simulink model "SVM_Stepper"  (R2020b)
settings: Solver=VariableStepAuto  StartTime=0.0  StopTime=1  FixedStep=0.0001  MaxStep=0.000005  RelTol=1e-3
values from neighbouring files (symbols this model uses):
  b = 0.05    [system_parameters.m]
  J = 48e-6    (= 4.8e-05)    [system_parameters.m]
  K_t = T_hold/I_rms    (= 0.575)    [system_parameters.m]
  L = 2e-3    (= 0.002)    [system_parameters.m]
  p = 50    [system_parameters.m]
  R = 0.5    [system_parameters.m]
  T_dm = 0.068    [system_parameters.m]
  T_load = 5.06e-3    (= 0.00506)    [system_parameters.m]
  U = 24    [system_parameters.m]
undefined symbols (not defined in the file or in its folder): Down, Up
libraries: fl_lib x90, ee_lib x55, eePwmGenerator x37, nesl_utility x33, dspsrcs4 x18, pid_lib x6, powerlib x4, eeDcCurrentController x1, eePmsmTorqueEstimator x1, simulink x1, eeQuadratureDecoder x1
(part 2 of 2)

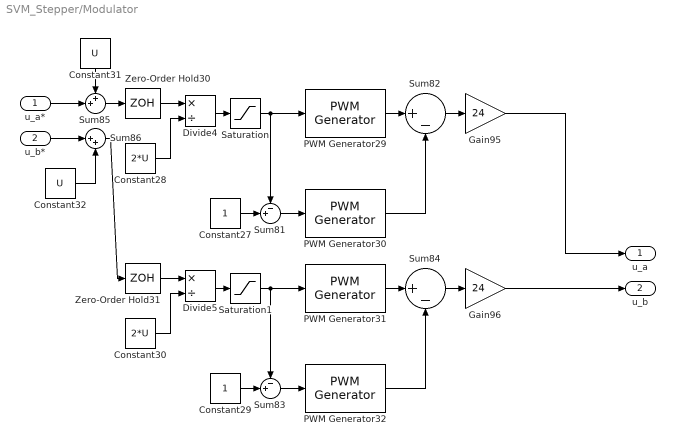
== system SVM_Stepper/Modulator ==
  u_a* : Inport
  u_b* : Inport  Port=2
  Constant27 : Constant
  Constant28 : Constant  Value=2*U
  Constant29 : Constant
  Constant30 : Constant  Value=2*U
  Constant31 : Constant  Value=U
  Constant32 : Constant  Value=U
  Divide4 : Product  Inputs=*/
  Divide5 : Product  Inputs=*/
  Gain95 : Gain  Gain=24
  Gain96 : Gain  Gain=24
  PWM Generator{29..32} (4 alike) : eePwmGenerator/PWM Generator  CarrCount=Up  Tper=25e-6  Ts=1e-6
  Saturation : Saturate  UpperLimit=1  LowerLimit=0
  Saturation1 : Saturate  UpperLimit=1  LowerLimit=0
  Sum81 : Sum  Inputs=-+|
  Sum82 : Sum  Inputs=|+-
  Sum83 : Sum  Inputs=-+|
  Sum84 : Sum  Inputs=|+-
  Sum85 : Sum  Inputs=++|
  Sum86 : Sum  Inputs=|++
  Zero-Order Hold30 : ZeroOrderHold  SampleTime=50e-6
  Zero-Order Hold31 : ZeroOrderHold  SampleTime=50e-6
  u_a : Outport
  u_b : Outport  Port=2
  wires:
  u_a*/1 -> Sum85/2
  Gain96/1 -> u_b/1
  Sum86/1 -> Zero-Order Hold31/1
  Saturation/1 -> PWM Generator29/1, Sum81/1
  Constant32/1 -> Sum86/2
  Zero-Order Hold30/1 -> Divide4/1
  Sum82/1 -> Gain95/1
  PWM Generator29/1 -> Sum82/1
  Constant30/1 -> Divide5/2
  Constant28/1 -> Divide4/2
  PWM Generator31/1 -> Sum84/1
  Saturation1/1 -> PWM Generator31/1, Sum83/1
  Divide4/1 -> Saturation/1
  PWM Generator30/1 -> Sum82/2
  Sum81/1 -> PWM Generator30/1
  Constant27/1 -> Sum81/2
  Constant29/1 -> Sum83/2
  Sum83/1 -> PWM Generator32/1
  Sum84/1 -> Gain96/1
  Divide5/1 -> Saturation1/1
  PWM Generator32/1 -> Sum84/2
  Zero-Order Hold31/1 -> Divide5/1
  Sum85/1 -> Zero-Order Hold30/1
  Constant31/1 -> Sum85/1
  Gain95/1 -> u_a/1
  u_b*/1 -> Sum86/1

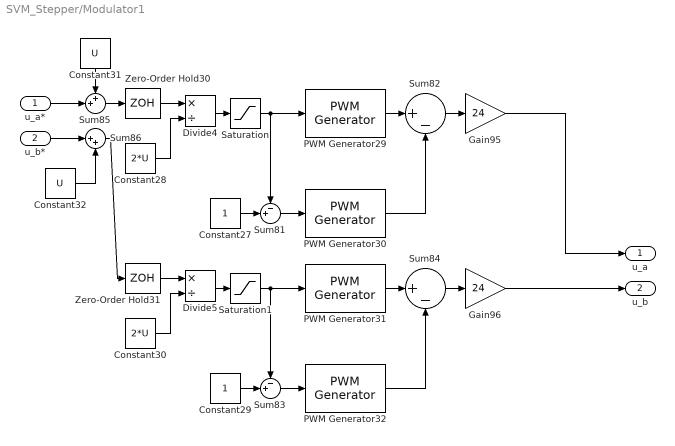
== system SVM_Stepper/Modulator1 ==
  u_a* : Inport
  u_b* : Inport  Port=2
  Constant27 : Constant
  Constant28 : Constant  Value=2*U
  Constant29 : Constant
  Constant30 : Constant  Value=2*U
  Constant31 : Constant  Value=U
  Constant32 : Constant  Value=U
  Divide4 : Product  Inputs=*/
  Divide5 : Product  Inputs=*/
  Gain95 : Gain  Gain=24
  Gain96 : Gain  Gain=24
  PWM Generator{29..32} (4 alike) : eePwmGenerator/PWM Generator  CarrCount=Up  Tper=25e-6  Ts=1e-6
  Saturation : Saturate  UpperLimit=1  LowerLimit=0
  Saturation1 : Saturate  UpperLimit=1  LowerLimit=0
  Sum81 : Sum  Inputs=-+|
  Sum82 : Sum  Inputs=|+-
  Sum83 : Sum  Inputs=-+|
  Sum84 : Sum  Inputs=|+-
  Sum85 : Sum  Inputs=++|
  Sum86 : Sum  Inputs=|++
  Zero-Order Hold30 : ZeroOrderHold  SampleTime=50e-6
  Zero-Order Hold31 : ZeroOrderHold  SampleTime=50e-6
  u_a : Outport
  u_b : Outport  Port=2
  wires:
  u_a*/1 -> Sum85/2
  Gain96/1 -> u_b/1
  Sum86/1 -> Zero-Order Hold31/1
  Saturation/1 -> PWM Generator29/1, Sum81/1
  Constant32/1 -> Sum86/2
  Zero-Order Hold30/1 -> Divide4/1
  Sum82/1 -> Gain95/1
  PWM Generator29/1 -> Sum82/1
  Constant30/1 -> Divide5/2
  Constant28/1 -> Divide4/2
  PWM Generator31/1 -> Sum84/1
  Saturation1/1 -> PWM Generator31/1, Sum83/1
  Divide4/1 -> Saturation/1
  PWM Generator30/1 -> Sum82/2
  Sum81/1 -> PWM Generator30/1
  Constant27/1 -> Sum81/2
  Constant29/1 -> Sum83/2
  Sum83/1 -> PWM Generator32/1
  Sum84/1 -> Gain96/1
  Divide5/1 -> Saturation1/1
  PWM Generator32/1 -> Sum84/2
  Zero-Order Hold31/1 -> Divide5/1
  Sum85/1 -> Zero-Order Hold30/1
  Constant31/1 -> Sum85/1
  Gain95/1 -> u_a/1
  u_b*/1 -> Sum86/1

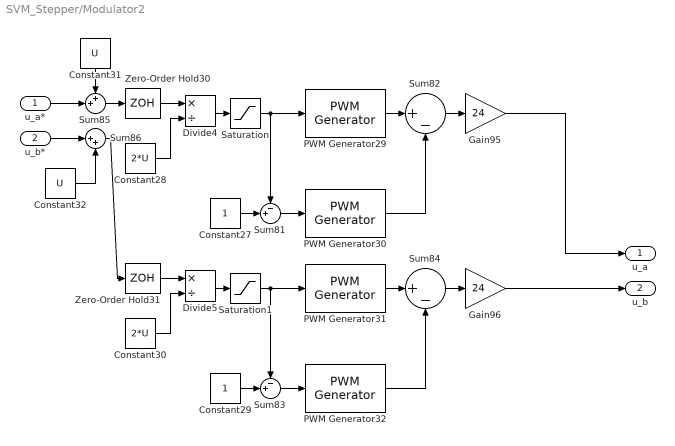
== system SVM_Stepper/Modulator2 ==
  u_a* : Inport
  u_b* : Inport  Port=2
  Constant27 : Constant
  Constant28 : Constant  Value=2*U
  Constant29 : Constant
  Constant30 : Constant  Value=2*U
  Constant31 : Constant  Value=U
  Constant32 : Constant  Value=U
  Divide4 : Product  Inputs=*/
  Divide5 : Product  Inputs=*/
  Gain95 : Gain  Gain=24
  Gain96 : Gain  Gain=24
  PWM Generator{29..32} (4 alike) : eePwmGenerator/PWM Generator  CarrCount=Up  Tper=25e-6  Ts=1e-6
  Saturation : Saturate  UpperLimit=1  LowerLimit=0
  Saturation1 : Saturate  UpperLimit=1  LowerLimit=0
  Sum81 : Sum  Inputs=-+|
  Sum82 : Sum  Inputs=|+-
  Sum83 : Sum  Inputs=-+|
  Sum84 : Sum  Inputs=|+-
  Sum85 : Sum  Inputs=++|
  Sum86 : Sum  Inputs=|++
  Zero-Order Hold30 : ZeroOrderHold  SampleTime=50e-6
  Zero-Order Hold31 : ZeroOrderHold  SampleTime=50e-6
  u_a : Outport
  u_b : Outport  Port=2
  wires:
  u_a*/1 -> Sum85/2
  Gain96/1 -> u_b/1
  Sum86/1 -> Zero-Order Hold31/1
  Saturation/1 -> PWM Generator29/1, Sum81/1
  Constant32/1 -> Sum86/2
  Zero-Order Hold30/1 -> Divide4/1
  Sum82/1 -> Gain95/1
  PWM Generator29/1 -> Sum82/1
  Constant30/1 -> Divide5/2
  Constant28/1 -> Divide4/2
  PWM Generator31/1 -> Sum84/1
  Saturation1/1 -> PWM Generator31/1, Sum83/1
  Divide4/1 -> Saturation/1
  PWM Generator30/1 -> Sum82/2
  Sum81/1 -> PWM Generator30/1
  Constant27/1 -> Sum81/2
  Constant29/1 -> Sum83/2
  Sum83/1 -> PWM Generator32/1
  Sum84/1 -> Gain96/1
  Divide5/1 -> Saturation1/1
  PWM Generator32/1 -> Sum84/2
  Zero-Order Hold31/1 -> Divide5/1
  Sum85/1 -> Zero-Order Hold30/1
  Constant31/1 -> Sum85/1
  Gain95/1 -> u_a/1
  u_b*/1 -> Sum86/1

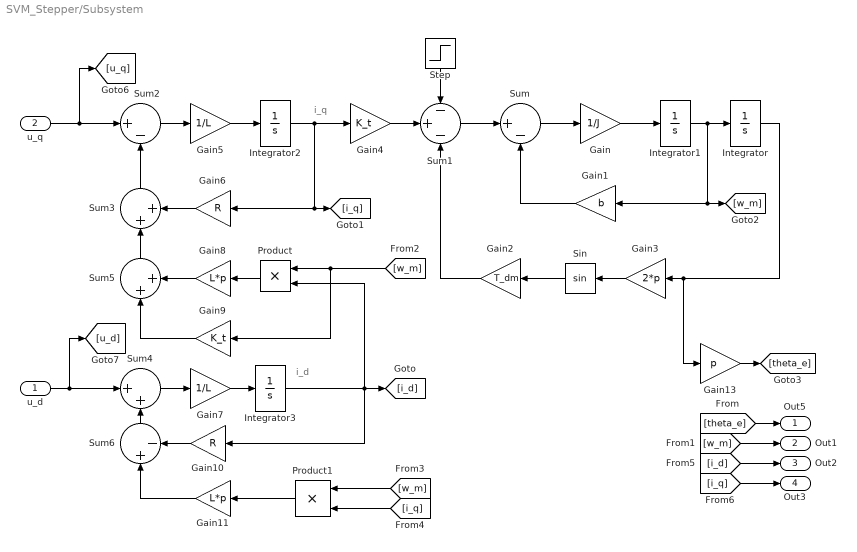
== system SVM_Stepper/Subsystem ==
  note: i_d
  note: i_q
  u_d : Inport
  u_q : Inport  Port=2
  Gain : Gain  Gain=1/J
  Gain1 : Gain  Gain=b
  Gain10 : Gain  Gain=R
  Gain11 : Gain  Gain=L*p
  Gain13 : Gain  Gain=p
  Gain2 : Gain  Gain=T_dm
  Gain3 : Gain  Gain=2*p
  Gain4 : Gain  Gain=K_t
  Gain5 : Gain  Gain=1/L
  Gain6 : Gain  Gain=R
  Gain7 : Gain  Gain=1/L
  Gain8 : Gain  Gain=L*p
  Gain9 : Gain  Gain=K_t
  Integrator{,1..3} (4 alike) : Integrator
  Product : Product
  Product1 : Product
  Sin : Trigonometry
  Step : Step  Time=7  After=T_load  SampleTime=0
  Sum : Sum  Inputs=|+-
  Sum1 : Sum  Inputs=-+-
  Sum2 : Sum  Inputs=|+-
  Sum3 : Sum  Inputs=|++
  Sum4 : Sum  Inputs=|++
  Sum5 : Sum  Inputs=|++
  Sum6 : Sum  Inputs=|+-
  Out5 : Outport
  Out1 : Outport  Port=2
  Out2 : Outport  Port=3
  Out3 : Outport  Port=4
  wires:
  Integrator/1 -> Gain13/1, Gain3/1
  Gain10/1 -> Sum6/2
  Gain6/1 -> Sum3/2
  Gain11/1 -> Sum6/1
  Gain1/1 -> Sum/2
  Sum/1 -> Gain/1
  Gain5/1 -> Integrator2/1
  Product/1 -> Gain8/1
  Integrator1/1 -> Gain1/1, [w_m], Integrator/1
  Integrator3/1 -> Gain10/1, Product/2, [i_d]
  Sum6/1 -> Sum4/2
  Sin/1 -> Gain2/1
  Integrator2/1 -> Gain4/1, Gain6/1, [i_q]
  Gain13/1 -> [theta_e]
  Sum5/1 -> Sum3/1
  Gain4/1 -> Sum1/2
  u_q/1 -> [u_q], Sum2/1
  u_d/1 -> [u_d], Sum4/1
  Product1/1 -> Gain11/1
  Sum3/1 -> Sum2/2
  Sum1/1 -> Sum/1
  Gain/1 -> Integrator1/1
  Gain2/1 -> Sum1/3
  [w_m] -> Product1/1
  Sum2/1 -> Gain5/1
  Gain3/1 -> Sin/1
  Gain7/1 -> Integrator3/1
  [i_q] -> Product1/2
  Gain9/1 -> Sum5/1
  Gain8/1 -> Sum5/2
  [w_m] -> Product/1, Gain9/1
  Step/1 -> Sum1/1
  Sum4/1 -> Gain7/1
  [theta_e] -> Out5/1
  [w_m] -> Out1/1
  [i_d] -> Out2/1
  [i_q] -> Out3/1

== matlab function SVM_Stepper/MATLAB Function6 ==
  data: X_a input; X_d output; X_b input; theta_e input; X_q output
function [X_d, X_q]= ForwardPark(X_a, X_b, theta_e)

    X_d = X_a*cos(theta_e) + X_b*sin(theta_e);
    X_q = -X_a*sin(theta_e) + X_b*cos(theta_e);

end

== matlab function SVM_Stepper/MATLAB Function7 ==
  data: X_q input; X_a output; X_d input; theta_e input; X_b output
function [X_a, X_b]= InversePark(X_q, X_d, theta_e)

    X_a = X_d*cos(theta_e) - X_q*sin(theta_e);
    X_b = X_d*sin(theta_e) + X_q*cos(theta_e);

end

== matlab function SVM_Stepper/MATLAB Function8 ==
  data: X_q input; X_a output; X_d input; theta_e input; X_b output
function [X_a, X_b]= InversePark(X_q, X_d, theta_e)

    X_a = X_d*cos(theta_e) - X_q*sin(theta_e);
    X_b = X_d*sin(theta_e) + X_q*cos(theta_e);

end

== matlab function SVM_Stepper/Two-phase SVM3 ==
  data: Ua input; DC_PWM1 output; Ub input; U input; Ts input; DC_PWM3 output; DC_PWM5 output; DC_PWM7 output
function [DC_PWM1, DC_PWM3, DC_PWM5, DC_PWM7] = fcn(Ua, Ub, U, Ts)

    V_r = sqrt(Ua^2 + Ub^2);
    if(V_r > U)
        V_r = U;
    end
    
    theta = atan2(Ub, Ua);
    if (theta < 0)
        theta = theta + 2*pi;
    end
    
    V1 = 0;     % Modulus of V1
    V2 = 0;     % Modulus of V2
%     VS = 0;
    theta_1 = 0;
    theta_2 = 0;
    
    sector = 0;
    
    if (theta >= 0 && theta < pi/4)
        % Sector I
        sector = 1;
        V1 = U;
        V2 = sqrt(2)*U;
        theta_1 = pi/4 - theta;
        theta_2 = theta;
    elseif (theta >= pi/4 && theta < pi/2)
        % Sector II
        sector = 2;
        V1 = U;
        V2 = sqrt(2)*U;
        theta_1 = theta - pi/4;
        theta_2 = pi/2 - theta;
    elseif (theta >= pi/2 && theta < 3*pi/4)
        % Sector III
        sector = 3;
        V1 = U;
        V2 = sqrt(2)*U;
        theta_1 = 3*pi/4 - theta;
        theta_2 = theta - pi/2;
    elseif (theta >= 3*pi/4 && theta < pi)
        % Sector IV
        sector = 4;
        V1 = U;
        V2 = sqrt(2)*U;
        theta_1 = theta - 3*pi/4;
        theta_2 = pi - theta;
    elseif (theta >= pi && theta < 5*pi/4)
        % Sector V
        sector = 5;
        V1 = U;
        V2 = sqrt(2)*U;
        theta_1 = 5*pi/4 - theta;
        theta_2 = theta - pi;
    elseif (theta >= 5*pi/4 && theta < 3*pi/2)
        % Sector VI
        sector = 6;
        V1 = U;
        V2 = sqrt(2)*U;
        theta_1 = theta - 5*pi/4;
        theta_2 = 3*pi/2 - theta;
    elseif (theta >= 3*pi/2 && theta < 7*pi/4)
        % Sector VII
        sector = 7;
        V1 = U;
        V2 = sqrt(2)*U;
        theta_1 = 7*pi/4 - theta;
        theta_2 = theta - 3*pi/2;
    elseif (theta >= 7*pi/4 && theta < 2*pi)
        % Sector VIII
        sector = 8;
        V1 = U;
        V2 = sqrt(2)*U;
        theta_1 = theta - 7*pi/4;
        theta_2 = 2*pi - theta;
    end

    T1 = Ts * (sqrt(2)*V_r/V1)*sin(theta_1);
    T2 = Ts * (sqrt(2)*V_r/V2)*sin(theta_2);
    
    TA = Ts;
    TB = Ts - T1 - T2;
    
    switch sector
        case 1
            DC_PWM1 = (TB + T1)/Ts;
            DC_PWM3 = 0;
            DC_PWM5 = TB/Ts;
            DC_PWM7 = 0;
        case 2
            DC_PWM1 = TB/Ts;
            DC_PWM3 = 0;
            DC_PWM5 = (TB + T1)/Ts;
            DC_PWM7 = 0;
        case 3
            DC_PWM1 = 0;
            DC_PWM3 = TB/Ts;
            DC_PWM5 =(TB + T1)/Ts;
            DC_PWM7 = 0; 
        case 4
            DC_PWM1 = 0;
            DC_PWM3 = (TB + T1)/Ts;
            DC_PWM5 = TB/Ts;
            DC_PWM7 = 0;
        case 5
            DC_PWM1 = 0;
            DC_PWM3 = (TB + T1)/Ts;
            DC_PWM5 = 0;
            DC_PWM7 = TB/Ts;
        case 6
            DC_PWM1 = 0;
            DC_PWM3 = TB/Ts;
            DC_PWM5 = 0;
            DC_PWM7 = (TB + T1)/Ts;
        case 7
            DC_PWM1 = TB/Ts;
            DC_PWM3 = 0;
            DC_PWM5 = 0;
            DC_PWM7 = (TB + T1)/Ts;
        case 8
            DC_PWM1 = (TB + T1)/Ts;
            DC_PWM3 = 0;
            DC_PWM5 = 0;
            DC_PWM7 = TB/Ts;
        otherwise
            DC_PWM1 = 0;
            DC_PWM3 = 0;
            DC_PWM5 = 0;
            DC_PWM7 = 0;
    end


end

== matlab function SVM_Stepper/Two-phase SVM2 ==
  data: Ua input; DC_PWM1 output; Ub input; U input; Ts input; DC_PWM3 output; DC_PWM5 output; DC_PWM7 output
function [DC_PWM1, DC_PWM3, DC_PWM5, DC_PWM7] = fcn(Ua, Ub, U, Ts)

    V_r = sqrt(Ua^2 + Ub^2);
    if(V_r > U)
        V_r = U;
    end
    
    theta = atan2(Ub, Ua);
    if (theta < 0)
        theta = theta + 2*pi;
    end
    
    V1 = 0;     % Modulus of V1
    V2 = 0;     % Modulus of V2
%     VS = 0;
    theta_1 = 0;
    theta_2 = 0;
    
    sector = 0;
    
    if (theta >= 0 && theta < pi/4)
        % Sector I
        sector = 1;
        V1 = U;
        V2 = sqrt(2)*U;
        theta_1 = pi/4 - theta;
        theta_2 = theta;
    elseif (theta >= pi/4 && theta < pi/2)
        % Sector II
        sector = 2;
        V1 = U;
        V2 = sqrt(2)*U;
        theta_1 = theta - pi/4;
        theta_2 = pi/2 - theta;
    elseif (theta >= pi/2 && theta < 3*pi/4)
        % Sector III
        sector = 3;
        V1 = U;
        V2 = sqrt(2)*U;
        theta_1 = 3*pi/4 - theta;
        theta_2 = theta - pi/2;
    elseif (theta >= 3*pi/4 && theta < pi)
        % Sector IV
        sector = 4;
        V1 = U;
        V2 = sqrt(2)*U;
        theta_1 = theta - 3*pi/4;
        theta_2 = pi - theta;
    elseif (theta >= pi && theta < 5*pi/4)
        % Sector V
        sector = 5;
        V1 = U;
        V2 = sqrt(2)*U;
        theta_1 = 5*pi/4 - theta;
        theta_2 = theta - pi;
    elseif (theta >= 5*pi/4 && theta < 3*pi/2)
        % Sector VI
        sector = 6;
        V1 = U;
        V2 = sqrt(2)*U;
        theta_1 = theta - 5*pi/4;
        theta_2 = 3*pi/2 - theta;
    elseif (theta >= 3*pi/2 && theta < 7*pi/4)
        % Sector VII
        sector = 7;
        V1 = U;
        V2 = sqrt(2)*U;
        theta_1 = 7*pi/4 - theta;
        theta_2 = theta - 3*pi/2;
    elseif (theta >= 7*pi/4 && theta < 2*pi)
        % Sector VIII
        sector = 8;
        V1 = U;
        V2 = sqrt(2)*U;
        theta_1 = theta - 7*pi/4;
        theta_2 = 2*pi - theta;
    end

    T1 = Ts * (sqrt(2)*V_r/V1)*sin(theta_1);
    T2 = Ts * (sqrt(2)*V_r/V2)*sin(theta_2);
    
    TA = Ts;
    TB = Ts - T1 - T2;
    
    switch sector
        case 1
            DC_PWM1 = (TB + T1)/Ts;
            DC_PWM3 = 0;
            DC_PWM5 = TB/Ts;
            DC_PWM7 = 0;
        case 2
            DC_PWM1 = TB/Ts;
            DC_PWM3 = 0;
            DC_PWM5 = (TB + T1)/Ts;
            DC_PWM7 = 0;
        case 3
            DC_PWM1 = 0;
            DC_PWM3 = TB/Ts;
            DC_PWM5 =(TB + T1)/Ts;
            DC_PWM7 = 0; 
        case 4
            DC_PWM1 = 0;
            DC_PWM3 = (TB + T1)/Ts;
            DC_PWM5 = TB/Ts;
            DC_PWM7 = 0;
        case 5
            DC_PWM1 = 0;
            DC_PWM3 = (TB + T1)/Ts;
            DC_PWM5 = 0;
            DC_PWM7 = TB/Ts;
        case 6
            DC_PWM1 = 0;
            DC_PWM3 = TB/Ts;
            DC_PWM5 = 0;
            DC_PWM7 = (TB + T1)/Ts;
        case 7
            DC_PWM1 = TB/Ts;
            DC_PWM3 = 0;
            DC_PWM5 = 0;
            DC_PWM7 = (TB + T1)/Ts;
        case 8
            DC_PWM1 = (TB + T1)/Ts;
            DC_PWM3 = 0;
            DC_PWM5 = 0;
            DC_PWM7 = TB/Ts;
        otherwise
            DC_PWM1 = 0;
            DC_PWM3 = 0;
            DC_PWM5 = 0;
            DC_PWM7 = 0;
    end


end

== matlab function SVM_Stepper/Two-phase SVM4 ==
  data: Ua input; DC_PWM1 output; Ub input; U input; Ts input; DC_PWM3 output; DC_PWM5 output; DC_PWM7 output
function [DC_PWM1, DC_PWM3, DC_PWM5, DC_PWM7] = fcn(Ua, Ub, U, Ts)

    V_r = sqrt(Ua^2 + Ub^2);
    if(V_r > U)
        V_r = U;
    end
    
    theta = atan2(Ub, Ua);
    if (theta < 0)
        theta = theta + 2*pi;
    end
    
    V1 = 0;     % Modulus of V1
    V2 = 0;     % Modulus of V2
%     VS = 0;
    theta_1 = 0;
    theta_2 = 0;
    
    sector = 0;
    
    if (theta >= 0 && theta < pi/4)
        % Sector I
        sector = 1;
        V1 = U;
        V2 = sqrt(2)*U;
        theta_1 = pi/4 - theta;
        theta_2 = theta;
    elseif (theta >= pi/4 && theta < pi/2)
        % Sector II
        sector = 2;
        V1 = U;
        V2 = sqrt(2)*U;
        theta_1 = theta - pi/4;
        theta_2 = pi/2 - theta;
    elseif (theta >= pi/2 && theta < 3*pi/4)
        % Sector III
        sector = 3;
        V1 = U;
        V2 = sqrt(2)*U;
        theta_1 = 3*pi/4 - theta;
        theta_2 = theta - pi/2;
    elseif (theta >= 3*pi/4 && theta < pi)
        % Sector IV
        sector = 4;
        V1 = U;
        V2 = sqrt(2)*U;
        theta_1 = theta - 3*pi/4;
        theta_2 = pi - theta;
    elseif (theta >= pi && theta < 5*pi/4)
        % Sector V
        sector = 5;
        V1 = U;
        V2 = sqrt(2)*U;
        theta_1 = 5*pi/4 - theta;
        theta_2 = theta - pi;
    elseif (theta >= 5*pi/4 && theta < 3*pi/2)
        % Sector VI
        sector = 6;
        V1 = U;
        V2 = sqrt(2)*U;
        theta_1 = theta - 5*pi/4;
        theta_2 = 3*pi/2 - theta;
    elseif (theta >= 3*pi/2 && theta < 7*pi/4)
        % Sector VII
        sector = 7;
        V1 = U;
        V2 = sqrt(2)*U;
        theta_1 = 7*pi/4 - theta;
        theta_2 = theta - 3*pi/2;
    elseif (theta >= 7*pi/4 && theta < 2*pi)
        % Sector VIII
        sector = 8;
        V1 = U;
        V2 = sqrt(2)*U;
        theta_1 = theta - 7*pi/4;
        theta_2 = 2*pi - theta;
    end

    T1 = Ts * (sqrt(2)*V_r/V1)*sin(theta_1);
    T2 = Ts * (sqrt(2)*V_r/V2)*sin(theta_2);
    
    TA = (Ts + T1 + T2)/2;
    TB = (Ts - T1 - T2)/2;
    

    switch sector
        case 1
            DC_PWM1 = TA;
            DC_PWM3 = TB;
            DC_PWM5 = TB + T1;
            DC_PWM7 = TB;
        case 2
            DC_PWM1 = TB + T1;
            DC_PWM3 = TB;
            DC_PWM5 = TA;
            DC_PWM7 = TB;
        case 3
            DC_PWM1 = TB;
            DC_PWM3 = TB + T1;
            DC_PWM5 = TA;
            DC_PWM7 = TB;
        case 4
            DC_PWM1 = TB;
            DC_PWM3 = TA;
            DC_PWM5 = TB + T1;
            DC_PWM7 = TB;
        case 5
            DC_PWM1 = TB;
            DC_PWM3 = TA;
            DC_PWM5 = TB;
            DC_PWM7 = TB + T1;
        case 6
            DC_PWM1 = TB;
            DC_PWM3 = TB + T1;
            DC_PWM5 = TB;
            DC_PWM7 = TA;
        case 7
            DC_PWM1 = TB + T1;
            DC_PWM3 = TB;
            DC_PWM5 = TB;
            DC_PWM7 = TA;
        case 8
            DC_PWM1 = TA;
            DC_PWM3 = TB;
            DC_PWM5 = TB;
            DC_PWM7 = TB + T1;
        otherwise
            DC_PWM1 = 0;
            DC_PWM3 = 0;
            DC_PWM5 = 0;
            DC_PWM7 = 0;
    end
    
    DC_PWM1 = DC_PWM1/Ts;
    DC_PWM3 = DC_PWM3/Ts;
    DC_PWM5 = DC_PWM5/Ts;
    DC_PWM7 = DC_PWM7/Ts;
end

== matlab function SVM_Stepper/MATLAB Function10 ==
  data: X_q input; X_a output; X_d input; theta_e input; X_b output
function [X_a, X_b]= InversePark(X_q, X_d, theta_e)

    X_a = X_d*cos(theta_e) - X_q*sin(theta_e);
    X_b = X_d*sin(theta_e) + X_q*cos(theta_e);

end

== matlab function SVM_Stepper/MATLAB Function9 ==
  data: X_q input; X_a output; X_d input; theta_e input; X_b output
function [X_a, X_b]= InversePark(X_q, X_d, theta_e)

    X_a = X_d*cos(theta_e) - X_q*sin(theta_e);
    X_b = X_d*sin(theta_e) + X_q*cos(theta_e);

end

== matlab function SVM_Stepper/MATLAB Function1 ==
  data: X_q input; X_a output; X_d input; theta_e input; X_b output
function [X_a, X_b]= InversePark(X_q, X_d, theta_e)

    X_a = X_d*cos(theta_e) - X_q*sin(theta_e);
    X_b = X_d*sin(theta_e) + X_q*cos(theta_e);

end

== matlab function SVM_Stepper/MATLAB Function11 ==
  data: X_q input; X_a output; X_d input; theta_e input; X_b output
function [X_a, X_b]= InversePark(X_q, X_d, theta_e)

    X_a = X_d*cos(theta_e) - X_q*sin(theta_e);
    X_b = X_d*sin(theta_e) + X_q*cos(theta_e);

end

== matlab function SVM_Stepper/MATLAB Function12 ==
  data: X_q input; X_a output; X_d input; theta_e input; X_b output
function [X_a, X_b]= InversePark(X_q, X_d, theta_e)

    X_a = X_d*cos(theta_e) - X_q*sin(theta_e);
    X_b = X_d*sin(theta_e) + X_q*cos(theta_e);

end

== matlab function SVM_Stepper/FCS MPC ==
  data: iq_ref input; Vq output; id_ref input; iq input; id input; omega_m input; theta_e input; Vcc input; Ts input; Vd output; R parameter; L parameter; p parameter; K_t parameter
function [Vq, Vd] = FCS_MPC(iq_ref, id_ref, iq, id, omega_m, theta_e, Vcc, Ts, R, L, p, K_t)

    Va_set = [Vcc, Vcc, 0, -Vcc, -Vcc, -Vcc, 0, Vcc, 0];
    Vb_set = [0, Vcc, Vcc, Vcc, 0, -Vcc, -Vcc, -Vcc, 0];
    
    cost = 1000;
    
    Vd = 0;
    Vq = 0;
    
    for i=1:9
        Va = Va_set(i);
        Vb = Vb_set(i);
        ud_current = Va*cos(theta_e) + Vb*sin(theta_e);
        uq_current = -Va*sin(theta_e)+ Vb*cos(theta_e);
       
        id_next = (1 - R*Ts/L)*id + Ts*p*omega_m*iq + (Ts/L)*ud_current;
        iq_next = (1 - R*Ts/L)*iq - Ts*p*omega_m*id + (Ts/L)*uq_current ...
            - Ts*K_t*omega_m/L;
        
        cost_current = (id_next - id_ref)^2 + (iq_next - iq_ref)^2;
        if (cost_current < cost)
            Vd = ud_current;
            Vq = uq_current;
            cost = cost_current;
        end
    end
    
end

== matlab function SVM_Stepper/MATLAB Function13 ==
  data: X_q input; X_a output; X_d input; theta_e input; X_b output
function [X_a, X_b]= InversePark(X_q, X_d, theta_e)

    X_a = X_d*cos(theta_e) - X_q*sin(theta_e);
    X_b = X_d*sin(theta_e) + X_q*cos(theta_e);

end

== matlab function SVM_Stepper/MATLAB Function14 ==
  data: X_q input; X_a output; X_d input; theta_e input; X_b output
function [X_a, X_b]= InversePark(X_q, X_d, theta_e)

    X_a = X_d*cos(theta_e) - X_q*sin(theta_e);
    X_b = X_d*sin(theta_e) + X_q*cos(theta_e);

end

== matlab function SVM_Stepper/MATLAB Function15 ==
  data: X_q input; X_a output; X_d input; theta_e input; X_b output
function [X_a, X_b]= InversePark(X_q, X_d, theta_e)

    X_a = X_d*cos(theta_e) - X_q*sin(theta_e);
    X_b = X_d*sin(theta_e) + X_q*cos(theta_e);

end

== matlab function SVM_Stepper/MATLAB Function16 ==
  data: X_a input; X_d output; X_b input; theta_e input; X_q output
function [X_d, X_q]= ForwardPark(X_a, X_b, theta_e)

    X_d = X_a*cos(theta_e) + X_b*sin(theta_e);
    X_q = -X_a*sin(theta_e) + X_b*cos(theta_e);

end

== matlab function SVM_Stepper/MATLAB Function17 ==
  data: X_q output; X_a input; X_d output; X_b input; theta_e input
function [X_q, X_d]= ForwardPark(X_a, X_b, theta_e)

    X_d = X_a*cos(theta_e) + X_b*sin(theta_e);
    X_q = -X_a*sin(theta_e) + X_b*cos(theta_e);

end

== matlab function SVM_Stepper/Deadbeat Control ==
  data: iq_ref input; Vq output; id_ref input; iq input; id input; omega_m input; theta_e input; Vcc input; Ts input; Vd output; R parameter; L parameter; p parameter; K_t parameter
function [Vq, Vd] = Deadbeat(iq_ref, id_ref, iq, id, omega_m, theta_e, Vcc, Ts, R, L, p, K_t)
% 
%     Va_set = [Vcc, Vcc, 0, -Vcc, -Vcc, -Vcc, 0, Vcc, 0];
%     Vb_set = [0, Vcc, Vcc, Vcc, 0, -Vcc, -Vcc, -Vcc, 0];
% %     
%     cost = 1000;
%     
    Vd = 0;
    Vq = 0;
    
    Vd = L*(id_ref - id)/Ts + R*id - p*L*iq*omega_m;
    Vq = L*(iq_ref - iq)/Ts + R*iq + p*L*id*omega_m + K_t*omega_m;
    
%     for i=1:9
%         Va = Va_set(i);
%         Vb = Vb_set(i);
%         ud_current = Va*cos(theta_e) + Vb*sin(theta_e);
%         uq_current = -Va*sin(theta_e)+ Vb*cos(theta_e);
%        
%         id_next = (1 - R*Ts/L)*id + Ts*p*omega_m*iq + (Ts/L)*ud_current;
%         iq_next = (1 - R*Ts/L)*iq - Ts*p*omega_m*id + (Ts/L)*uq_current ...
%             - Ts*K_t*omega_m/L;
%         
%         cost_current = (id_next - id_ref)^2 + (iq_next - iq_ref)^2;
%         if (cost_current < cost)
%             Vd = ud_current;
%             Vq = uq_current;
%             cost = cost_current;
%         end
%     end
    
end

== matlab function SVM_Stepper/MATLAB Function ==
  data: X_a input; X_d output; X_b input; theta_e input; X_q output
function [X_d, X_q]= ForwardPark(X_a, X_b, theta_e)

    X_d = X_a*cos(theta_e) + X_b*sin(theta_e);
    X_q = -X_a*sin(theta_e) + X_b*cos(theta_e);

end

== matlab function SVM_Stepper/MATLAB Function18 ==
  data: X_q input; X_a output; X_d input; theta_e input; X_b output
function [X_a, X_b]= InversePark(X_q, X_d, theta_e)

    X_a = X_d*cos(theta_e) - X_q*sin(theta_e);
    X_b = X_d*sin(theta_e) + X_q*cos(theta_e);

end

== matlab function SVM_Stepper/MATLAB Function19 ==
  data: X_q input; X_a output; X_d input; theta_e input; X_b output
function [X_a, X_b]= InversePark(X_q, X_d, theta_e)

    X_a = X_d*cos(theta_e) - X_q*sin(theta_e);
    X_b = X_d*sin(theta_e) + X_q*cos(theta_e);

end

== matlab function SVM_Stepper/MATLAB Function20 ==
  data: X_q input; X_a output; X_d input; theta_e input; X_b output
function [X_a, X_b]= InversePark(X_q, X_d, theta_e)

    X_a = X_d*cos(theta_e) - X_q*sin(theta_e);
    X_b = X_d*sin(theta_e) + X_q*cos(theta_e);

end

== matlab function SVM_Stepper/MATLAB Function21 ==
  data: X_q output; X_a input; X_d output; X_b input; theta_e input
function [X_q, X_d]= ForwardPark(X_a, X_b, theta_e)

    X_d = X_a*cos(theta_e) + X_b*sin(theta_e);
    X_q = -X_a*sin(theta_e) + X_b*cos(theta_e);

end

== matlab function SVM_Stepper/Deadbeat Control1 ==
  data: iq_ref input; Vq output; id_ref input; iq input; id input; omega_m input; theta_e input; Vcc input; Ts input; Vd output; R parameter; L parameter; p parameter; K_t parameter
function [Vq, Vd] = Deadbeat(iq_ref, id_ref, iq, id, omega_m, theta_e, Vcc, Ts, R, L, p, K_t)
% 
%     Va_set = [Vcc, Vcc, 0, -Vcc, -Vcc, -Vcc, 0, Vcc, 0];
%     Vb_set = [0, Vcc, Vcc, Vcc, 0, -Vcc, -Vcc, -Vcc, 0];
% %     
%     cost = 1000;
%     
    Vd = 0;
    Vq = 0;
    
    Vd = L*(id_ref - id)/Ts + R*id - p*L*iq*omega_m;
    Vq = L*(iq_ref - iq)/Ts + R*iq + p*L*id*omega_m + K_t*omega_m;
    
%     for i=1:9
%         Va = Va_set(i);
%         Vb = Vb_set(i);
%         ud_current = Va*cos(theta_e) + Vb*sin(theta_e);
%         uq_current = -Va*sin(theta_e)+ Vb*cos(theta_e);
%        
%         id_next = (1 - R*Ts/L)*id + Ts*p*omega_m*iq + (Ts/L)*ud_current;
%         iq_next = (1 - R*Ts/L)*iq - Ts*p*omega_m*id + (Ts/L)*uq_current ...
%             - Ts*K_t*omega_m/L;
%         
%         cost_current = (id_next - id_ref)^2 + (iq_next - iq_ref)^2;
%         if (cost_current < cost)
%             Vd = ud_current;
%             Vq = uq_current;
%             cost = cost_current;
%         end
%     end
    
end

== matlab function SVM_Stepper/FCS MPC1 ==
  data: iq_ref input; Vq output; id_ref input; iq input; id input; omega_m input; theta_e input; Vcc input; Ts input; Vd output; R parameter; L parameter; p parameter; K_t parameter
function [Vq, Vd] = FCS_MPC(iq_ref, id_ref, iq, id, omega_m, theta_e, Vcc, Ts, R, L, p, K_t)

    Va_set = [Vcc, Vcc, 0, -Vcc, -Vcc, -Vcc, 0, Vcc, 0];
    Vb_set = [0, Vcc, Vcc, Vcc, 0, -Vcc, -Vcc, -Vcc, 0];
    
    cost = 1000;
    
    Vd = 0;
    Vq = 0;
    
    for i=1:9
        Va = Va_set(i);
        Vb = Vb_set(i);
        ud_current = Va*cos(theta_e) + Vb*sin(theta_e);
        uq_current = -Va*sin(theta_e)+ Vb*cos(theta_e);
       
        id_next = (1 - R*Ts/L)*id + Ts*p*omega_m*iq + (Ts/L)*ud_current;
        iq_next = (1 - R*Ts/L)*iq - Ts*p*omega_m*id + (Ts/L)*uq_current ...
            - Ts*K_t*omega_m/L;
        
        cost_current = (id_next - id_ref)^2 + (iq_next - iq_ref)^2;
        if (cost_current < cost)
            Vd = ud_current;
            Vq = uq_current;
            cost = cost_current;
        end
    end
    
end

== matlab function SVM_Stepper/MATLAB Function24 ==
  data: X_q input; X_a output; X_d input; theta_e input; X_b output
function [X_a, X_b]= InversePark(X_q, X_d, theta_e)

    X_a = X_d*cos(theta_e) - X_q*sin(theta_e);
    X_b = X_d*sin(theta_e) + X_q*cos(theta_e);

end

== matlab function SVM_Stepper/MATLAB Function2 ==
  data: X_q input; X_a output; X_d input; theta_e input; X_b output
function [X_a, X_b]= InversePark(X_q, X_d, theta_e)

    X_a = X_d*cos(theta_e) - X_q*sin(theta_e);
    X_b = X_d*sin(theta_e) + X_q*cos(theta_e);

end

== matlab function SVM_Stepper/MATLAB Function25 ==
  data: X_q output; X_a input; X_d output; X_b input; theta_e input
function [X_q, X_d]= ForwardPark(X_a, X_b, theta_e)

    X_d = X_a*cos(theta_e) + X_b*sin(theta_e);
    X_q = -X_a*sin(theta_e) + X_b*cos(theta_e);

end

== matlab function SVM_Stepper/MATLAB Function3 ==
  data: X_q input; X_a output; X_d input; theta_e input; X_b output
function [X_a, X_b]= InversePark(X_q, X_d, theta_e)

    X_a = X_d*cos(theta_e) - X_q*sin(theta_e);
    X_b = X_d*sin(theta_e) + X_q*cos(theta_e);

end

== matlab function SVM_Stepper/Two-phase SVM ==
  data: Ua input; DC_PWM1 output; Ub input; U input; Ts input; DC_PWM3 output; DC_PWM5 output; DC_PWM7 output
function [DC_PWM1, DC_PWM3, DC_PWM5, DC_PWM7] = fcn(Ua, Ub, U, Ts)

    V_r = sqrt(Ua^2 + Ub^2);
    if(V_r > U)
        V_r = U;
    end
    
    theta = atan2(Ub, Ua);
    if (theta < 0)
        theta = theta + 2*pi;
    end
    
    V1 = 0;     % Modulus of V1
    V2 = 0;     % Modulus of V2
%     VS = 0;
    theta_1 = 0;
    theta_2 = 0;
    
    sector = 0;
    
    if (theta >= 0 && theta < pi/4)
        % Sector I
        sector = 1;
        V1 = U;
        V2 = sqrt(2)*U;
        theta_1 = pi/4 - theta;
        theta_2 = theta;
    elseif (theta >= pi/4 && theta < pi/2)
        % Sector II
        sector = 2;
        V1 = U;
        V2 = sqrt(2)*U;
        theta_1 = theta - pi/4;
        theta_2 = pi/2 - theta;
    elseif (theta >= pi/2 && theta < 3*pi/4)
        % Sector III
        sector = 3;
        V1 = U;
        V2 = sqrt(2)*U;
        theta_1 = 3*pi/4 - theta;
        theta_2 = theta - pi/2;
    elseif (theta >= 3*pi/4 && theta < pi)
        % Sector IV
        sector = 4;
        V1 = U;
        V2 = sqrt(2)*U;
        theta_1 = theta - 3*pi/4;
        theta_2 = pi - theta;
    elseif (theta >= pi && theta < 5*pi/4)
        % Sector V
        sector = 5;
        V1 = U;
        V2 = sqrt(2)*U;
        theta_1 = 5*pi/4 - theta;
        theta_2 = theta - pi;
    elseif (theta >= 5*pi/4 && theta < 3*pi/2)
        % Sector VI
        sector = 6;
        V1 = U;
        V2 = sqrt(2)*U;
        theta_1 = theta - 5*pi/4;
        theta_2 = 3*pi/2 - theta;
    elseif (theta >= 3*pi/2 && theta < 7*pi/4)
        % Sector VII
        sector = 7;
        V1 = U;
        V2 = sqrt(2)*U;
        theta_1 = 7*pi/4 - theta;
        theta_2 = theta - 3*pi/2;
    elseif (theta >= 7*pi/4 && theta < 2*pi)
        % Sector VIII
        sector = 8;
        V1 = U;
        V2 = sqrt(2)*U;
        theta_1 = theta - 7*pi/4;
        theta_2 = 2*pi - theta;
    end

    T1 = Ts * (sqrt(2)*V_r/V1)*sin(theta_1);
    T2 = Ts * (sqrt(2)*V_r/V2)*sin(theta_2);
    
    TA = Ts;
    TB = Ts - T1 - T2;
    
    switch sector
        case 1
            DC_PWM1 = (TB + T1)/Ts;
            DC_PWM3 = 0;
            DC_PWM5 = TB/Ts;
            DC_PWM7 = 0;
        case 2
            DC_PWM1 = TB/Ts;
            DC_PWM3 = 0;
            DC_PWM5 = (TB + T1)/Ts;
            DC_PWM7 = 0;
        case 3
            DC_PWM1 = 0;
            DC_PWM3 = TB/Ts;
            DC_PWM5 =(TB + T1)/Ts;
            DC_PWM7 = 0; 
        case 4
            DC_PWM1 = 0;
            DC_PWM3 = (TB + T1)/Ts;
            DC_PWM5 = TB/Ts;
            DC_PWM7 = 0;
        case 5
            DC_PWM1 = 0;
            DC_PWM3 = (TB + T1)/Ts;
            DC_PWM5 = 0;
            DC_PWM7 = TB/Ts;
        case 6
            DC_PWM1 = 0;
            DC_PWM3 = TB/Ts;
            DC_PWM5 = 0;
            DC_PWM7 = (TB + T1)/Ts;
        case 7
            DC_PWM1 = TB/Ts;
            DC_PWM3 = 0;
            DC_PWM5 = 0;
            DC_PWM7 = (TB + T1)/Ts;
        case 8
            DC_PWM1 = (TB + T1)/Ts;
            DC_PWM3 = 0;
            DC_PWM5 = 0;
            DC_PWM7 = TB/Ts;
        otherwise
            DC_PWM1 = 0;
            DC_PWM3 = 0;
            DC_PWM5 = 0;
            DC_PWM7 = 0;
    end


end

== matlab function SVM_Stepper/Two-phase SVM1 ==
  data: Ua input; DC_PWM1 output; Ub input; U input; Ts input; DC_PWM3 output; DC_PWM5 output; DC_PWM7 output
function [DC_PWM1, DC_PWM3, DC_PWM5, DC_PWM7] = fcn(Ua, Ub, U, Ts)

    V_r = sqrt(Ua^2 + Ub^2);
    if(V_r > U)
        V_r = U;
    end
    
    theta = atan2(Ub, Ua);
    if (theta < 0)
        theta = theta + 2*pi;
    end
    
    V1 = 0;     % Modulus of V1
    V2 = 0;     % Modulus of V2
%     VS = 0;
    theta_1 = 0;
    theta_2 = 0;
    
    sector = 0;
    
    if (theta >= 0 && theta < pi/4)
        % Sector I
        sector = 1;
        V1 = U;
        V2 = sqrt(2)*U;
        theta_1 = pi/4 - theta;
        theta_2 = theta;
    elseif (theta >= pi/4 && theta < pi/2)
        % Sector II
        sector = 2;
        V1 = U;
        V2 = sqrt(2)*U;
        theta_1 = theta - pi/4;
        theta_2 = pi/2 - theta;
    elseif (theta >= pi/2 && theta < 3*pi/4)
        % Sector III
        sector = 3;
        V1 = U;
        V2 = sqrt(2)*U;
        theta_1 = 3*pi/4 - theta;
        theta_2 = theta - pi/2;
    elseif (theta >= 3*pi/4 && theta < pi)
        % Sector IV
        sector = 4;
        V1 = U;
        V2 = sqrt(2)*U;
        theta_1 = theta - 3*pi/4;
        theta_2 = pi - theta;
    elseif (theta >= pi && theta < 5*pi/4)
        % Sector V
        sector = 5;
        V1 = U;
        V2 = sqrt(2)*U;
        theta_1 = 5*pi/4 - theta;
        theta_2 = theta - pi;
    elseif (theta >= 5*pi/4 && theta < 3*pi/2)
        % Sector VI
        sector = 6;
        V1 = U;
        V2 = sqrt(2)*U;
        theta_1 = theta - 5*pi/4;
        theta_2 = 3*pi/2 - theta;
    elseif (theta >= 3*pi/2 && theta < 7*pi/4)
        % Sector VII
        sector = 7;
        V1 = U;
        V2 = sqrt(2)*U;
        theta_1 = 7*pi/4 - theta;
        theta_2 = theta - 3*pi/2;
    elseif (theta >= 7*pi/4 && theta < 2*pi)
        % Sector VIII
        sector = 8;
        V1 = U;
        V2 = sqrt(2)*U;
        theta_1 = theta - 7*pi/4;
        theta_2 = 2*pi - theta;
    end

    T1 = Ts * (sqrt(2)*V_r/V1)*sin(theta_1);
    T2 = Ts * (sqrt(2)*V_r/V2)*sin(theta_2);
    
    TA = Ts;
    TB = Ts - T1 - T2;
    
    switch sector
        case 1
            DC_PWM1 = (TB + T1)/Ts;
            DC_PWM3 = 0;
            DC_PWM5 = TB/Ts;
            DC_PWM7 = 0;
        case 2
            DC_PWM1 = TB/Ts;
            DC_PWM3 = 0;
            DC_PWM5 = (TB + T1)/Ts;
            DC_PWM7 = 0;
        case 3
            DC_PWM1 = 0;
            DC_PWM3 = TB/Ts;
            DC_PWM5 =(TB + T1)/Ts;
            DC_PWM7 = 0; 
        case 4
            DC_PWM1 = 0;
            DC_PWM3 = (TB + T1)/Ts;
            DC_PWM5 = TB/Ts;
            DC_PWM7 = 0;
        case 5
            DC_PWM1 = 0;
            DC_PWM3 = (TB + T1)/Ts;
            DC_PWM5 = 0;
            DC_PWM7 = TB/Ts;
        case 6
            DC_PWM1 = 0;
            DC_PWM3 = TB/Ts;
            DC_PWM5 = 0;
            DC_PWM7 = (TB + T1)/Ts;
        case 7
            DC_PWM1 = TB/Ts;
            DC_PWM3 = 0;
            DC_PWM5 = 0;
            DC_PWM7 = (TB + T1)/Ts;
        case 8
            DC_PWM1 = (TB + T1)/Ts;
            DC_PWM3 = 0;
            DC_PWM5 = 0;
            DC_PWM7 = TB/Ts;
        otherwise
            DC_PWM1 = 0;
            DC_PWM3 = 0;
            DC_PWM5 = 0;
            DC_PWM7 = 0;
    end


end

== matlab function SVM_Stepper/MATLAB Function4 ==
  data: X_q input; X_a output; X_d input; theta_e input; X_b output
function [X_a, X_b]= InversePark(X_q, X_d, theta_e)

    X_a = X_d*cos(theta_e) - X_q*sin(theta_e);
    X_b = X_d*sin(theta_e) + X_q*cos(theta_e);

end

== matlab function SVM_Stepper/MATLAB Function5 ==
  data: X_a input; X_d output; X_b input; theta_e input; X_q output
function [X_d, X_q]= ForwardPark(X_a, X_b, theta_e)

    X_d = X_a*cos(theta_e) + X_b*sin(theta_e);
    X_q = -X_a*sin(theta_e) + X_b*cos(theta_e);

end
